simulink model "Cardio_SA_LV_EarlyVersion"  (R2021a)
settings: Solver=ode1  StartTime=0.0  StopTime=Beats  FixedStep=dt  MinStep=.001  RelTol=1e-3  EnableMultiTasking=on
PreLoadFcn:
  | %Time parameters
  | T = 0.0125;   %Duration of heartbeat (minutes)
  | Ts = 0.0050;   %Duration of systole   (minutes)
  | Stroke_volume = 70e-3;
  | Tmax = 0.0020;  %Time at which flow is max (minutes)
  | Qmax= Stroke_volume/(0.5*Ts);    %Max flow through aortic valve (liters/minute)
  | dt = .00005*T;
  | %This choice implies 20,000 timesteps per cardiac cycle
  | 
  | %Compliance and resistance parameters. Note that valve resistances are not
  | %supposed to be realistic, just small enough to be negligible
  | Csa = .00175; %Systemic arterial compliance (liters/(mmHg))
  | Rs = 17.86; %Systemic resistance (mmHg/(liters/minute))
  | Rmi = .01; %mitral valve resistance (mmHg/(liters/minute))
  | RAo = .01; %Aortic valve resistance (mmHg/(liters/minute))
  | 
  | Vlvd = .027; %Left ventricular volume when PLV = 0 (liters)
  | Vsad = .825; %Systemic arterial volume when Psa = 0 (liters)
  | Pla = 5; %Left atrial pressure (mmHg)
  | 
  | %Parameters for Clv(t)
  | CLVD = .0146; %Max (diastolic) value of CLV (liters/mmHg)
  | CLVS = .00003; %Min (systolic) value of CLV (liters/mmHg)
  | tauS = .0025; %CLV time constant during systole (minutes)
  | tauD = .001; %CLV time constant during diastole (minutes)
  | 
  | %Initialization parameters
  | Plvi = 5; %initial value of PLV (mmHg)
  | Psai = 80; %initial value of Psa (mmHg)
  | 
  | %Don't forget to plot VSA vs. PSA and VLV vs. PLV!!!!!!! The values have
  | %been exported into the matlab workspace so you can plot them yourself!
values from neighbouring files (symbols this model uses):
  AoBkflo = 0.00    (= 0)    [Command_Cardio_SA_LV.m]
settings Model: Creator=MRFIL  LastModifiedBy=claudelieber
settings SolverCC: AlgebraicLoopSolver=TrustRegion
settings DataIOCC: LimitDataPoints=on  SaveFormat=Array  SignalLoggingSaveFormat=ModelDataLogs  ReturnWorkspaceOutputs=off
settings OptimizationCC: ExpressionDepthLimit=2147483647  LifeSpan=inf
settings DebuggingCC: UnderspecifiedInitializationDetection=Classic  MergeDetectMultiDrivingBlocksExec=none  SolverPrmCheckMsg=warning  FcnCallInpInsideContextMsg=warning  StateNameClashWarn=warning  SFUnexpectedBacktrackingDiag=warning  SFNoUnconditionalDefaultTransitionDiag=warning  SFExecutionAtInitializationDiag=none  ArithmeticOperatorsInVariantConditions=warning
settings HardwareCC: ProdBitPerPointer=32  ProdBitPerSizeT=32  ProdBitPerPtrDiffT=32  ProdLargestAtomicFloat=None  ProdIntDivRoundTo=Undefined  ProdEndianess=Unspecified  ProdWordSize=32  ProdHWDeviceType=32-bit Generic
settings ModelReferenceCC: PropagateSignalLabelsOutOfModel=off
settings SFSimCC: SimUseLocalCustomCode=off  CustomCodeUndefinedFunction=UseInterfaceOnly
settings RTWCC: RTWUseLocalCustomCode=off  DLArmComputeVersion=20.02.1
settings CodeAppCC: StateflowObjectComments=on
settings GRTTargetCC: TargetLangStandard=C89/C90 (ANSI)  CombineOutputUpdateFcns=off  GRTInterface=on
settings ConfigComp: CovMetricSettings=dw  CovSaveCumulativeToWorkspaceVar=on  CovSaveSingleToWorkspaceVar=on  CovExternalEMLEnable=off

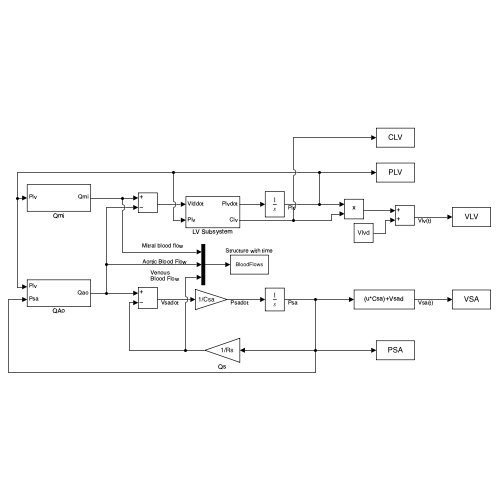
[thumbnail: Simulink's stored preview of the top-level diagram]
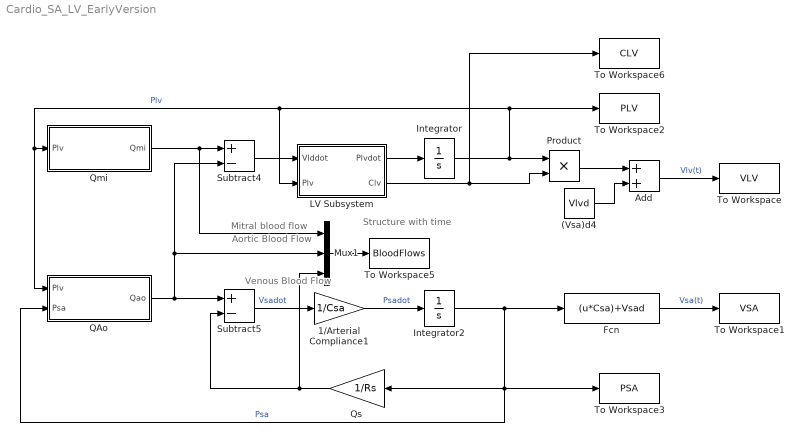
== system Cardio_SA_LV_EarlyVersion ==
  note: Structure with time
  note: Venous
      | Blood Flow
  note: Aortic Blood Flow
  note: Mitral blood flow
  (Vsa)d4 : Constant  Value=Vlvd
  1/Arterial Compliance1 : Gain  Gain=1/Csa
  Add : Sum
  Fcn : Fcn  Expr=(u*Csa)+Vsad
  Integrator : Integrator  InitialCondition=Plvi
  Integrator2 : Integrator  InitialCondition=Psai
  LV Subsystem : Subsystem
  Mux1 : Mux  Inputs=3
  Product : Product  RndMeth=Zero
  QAo : Subsystem
  Qmi : Subsystem
  Qs : Gain  Gain=1/Rs
  Subtract4 : Sum  Inputs=+-
  Subtract5 : Sum  Inputs=+-
  To Workspace : ToWorkspace  VariableName=VLV  SampleTime=-1
  To Workspace1 : ToWorkspace  VariableName=VSA  SampleTime=-1
  To Workspace2 : ToWorkspace  VariableName=PLV  SampleTime=-1
  To Workspace3 : ToWorkspace  VariableName=PSA  SampleTime=-1
  To Workspace5 : ToWorkspace  VariableName=BloodFlows  SaveFormat=Structure With Time  SampleTime=-1
  To Workspace6 : ToWorkspace  VariableName=CLV  SampleTime=-1
  wires:
  Fcn/1 -> To Workspace1/1  "Vsa(t)"
  Subtract5/1 -> 1/Arterial Compliance1/1  "Vsadot"
  1/Arterial Compliance1/1 -> Integrator2/1  "Psadot"
  Integrator2/1 -> QAo/2(Psa), To Workspace3/1, Qs/1, Fcn/1  "Psa"
  Qs/1 -> Subtract5/2, Mux1/3
  QAo/1(Qao) -> Mux1/2, Subtract4/2, Subtract5/1
  Qmi/1(Qmi) -> Subtract4/1, Mux1/1
  Product/1 -> Add/1
  (Vsa)d4/1 -> Add/2
  Add/1 -> To Workspace/1  "Vlv(t)"
  Subtract4/1 -> LV Subsystem/1(Vlddot)
  LV Subsystem/1(Plvdot) -> Integrator/1
  Integrator/1 -> Product/1, LV Subsystem/2(Plv), QAo/1(Plv), Qmi/1(Plv), To Workspace2/1  "Plv"
  LV Subsystem/2(Clv) -> To Workspace6/1, Product/2
  Mux1/1 -> To Workspace5/1

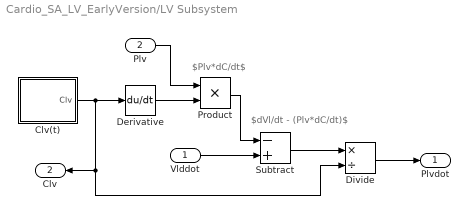
== system Cardio_SA_LV_EarlyVersion/LV Subsystem ==
  note: $dVl/dt - (Plv*dC/dt)$
  note: $Plv*dC/dt$
  Vlddot : Inport
  Plv : Inport  Port=2
  Clv(t) : Subsystem
  Derivative : Derivative
  Divide : Product  Inputs=*/
  Product : Product  RndMeth=Zero
  Subtract : Sum  Inputs=-+
  Plvdot : Outport  VectorParamsAs1DForOutWhenUnconnected=off
  Clv : Outport  Port=2  VectorParamsAs1DForOutWhenUnconnected=off
  wires:
  Clv(t)/1(Clv) -> Derivative/1, Clv/1, Divide/2
  Derivative/1 -> Product/2
  Plv/1 -> Product/1
  Product/1 -> Subtract/1
  Vlddot/1 -> Subtract/2
  Subtract/1 -> Divide/1
  Divide/1 -> Plvdot/1

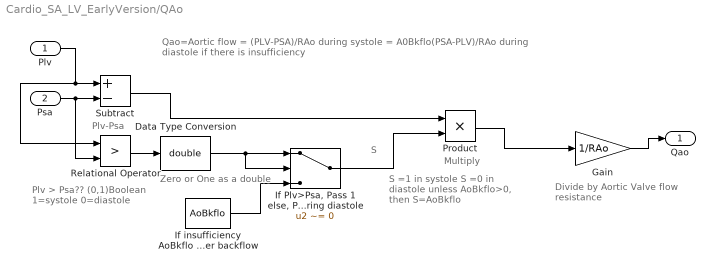
== system Cardio_SA_LV_EarlyVersion/QAo ==
  note: S
  note: S =1 in systole
      | S =0 in diastole
      | unless AoBkflo>0,
      | then S=AoBkflo
  note: Qao=Aortic flow = (PLV-PSA)/RAo during systole
      | = A0Bkflo(PSA-PLV)/RAo during diastole
      | if there is insufficiency
  note: Divide by
      | Aortic Valve
      | flow resistance
  note: Plv > Psa??
      | (0,1)Boolean
      | 1=systole
      | 0=diastole
  note: Multiply
  note: Zero or One
      | as a double
  note: Plv-Psa
  Plv : Inport
  Psa : Inport  Port=2
  Data Type Conversion : DataTypeConversion  OutDataTypeStr=double
  Gain : Gain  Gain=1/RAo
  "If Plv>Psa, Pass 1 else, Pass AoBkflo i.e. pass PLV-PSA during systole and AoBkflo*(PSA-PLV) during diastole" : Switch  Criteria=u2 ~= 0
  If insufficiency AoBkflo multiplies pressure difference during diastole divided by RAo to render backflow : Constant  Value=AoBkflo
  Product : Product  RndMeth=Zero
  Relational Operator : RelationalOperator  Operator=>  OutDataTypeStr=boolean  RndMeth=Nearest
  Subtract : Sum  Inputs=+-
  Qao : Outport  VectorParamsAs1DForOutWhenUnconnected=off
  wires:
  "If Plv>Psa, Pass 1 else, Pass AoBkflo i.e. pass PLV-PSA during systole and AoBkflo*(PSA-PLV) during diastole"/1 -> Product/2
  Relational Operator/1 -> Data Type Conversion/1
  Gain/1 -> Qao/1
  Psa/1 -> Subtract/2, Relational Operator/2
  Product/1 -> Gain/1
  Data Type Conversion/1 -> "If Plv>Psa, Pass 1 else, Pass AoBkflo i.e. pass PLV-PSA during systole and AoBkflo*(PSA-PLV) during diastole"/2, "If Plv>Psa, Pass 1 else, Pass AoBkflo i.e. pass PLV-PSA during systole and AoBkflo*(PSA-PLV) during diastole"/1
  If insufficiency AoBkflo multiplies pressure difference during diastole divided by RAo to render backflow/1 -> "If Plv>Psa, Pass 1 else, Pass AoBkflo i.e. pass PLV-PSA during systole and AoBkflo*(PSA-PLV) during diastole"/3
  Plv/1 -> Subtract/1, Relational Operator/1
  Subtract/1 -> Product/1

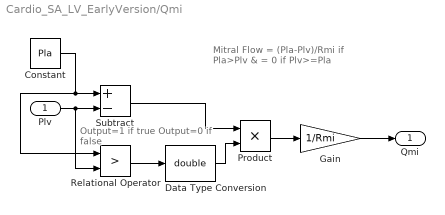
== system Cardio_SA_LV_EarlyVersion/Qmi ==
  note: Mitral Flow = (Pla-Plv)/Rmi if Pla>Plv
      | & = 0 if Plv>=Pla
  note: Output=1 if true
      | Output=0 if false
  Plv : Inport
  Constant : Constant  Value=Pla
  Data Type Conversion : DataTypeConversion  OutDataTypeStr=double
  Gain : Gain  Gain=1/Rmi
  Product : Product  RndMeth=Zero
  Relational Operator : RelationalOperator  Operator=>  OutDataTypeStr=boolean  RndMeth=Nearest
  Subtract : Sum  Inputs=+-
  Qmi : Outport  VectorParamsAs1DForOutWhenUnconnected=off
  wires:
  Constant/1 -> Relational Operator/1, Subtract/1
  Subtract/1 -> Product/1
  Product/1 -> Gain/1
  Gain/1 -> Qmi/1
  Plv/1 -> Relational Operator/2, Subtract/2
  Data Type Conversion/1 -> Product/2
  Relational Operator/1 -> Data Type Conversion/1

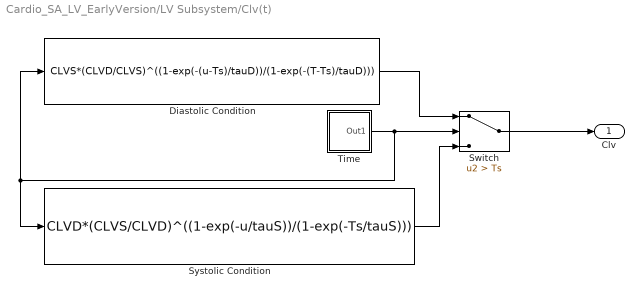
== system Cardio_SA_LV_EarlyVersion/LV Subsystem/Clv(t) ==
  Diastolic Condition : Fcn  Expr=CLVS*(CLVD/CLVS)^((1-exp(-(u-Ts)/tauD))/(1-exp(-(T-Ts)/tauD)))
  Switch : Switch  Criteria=u2 > Threshold  Threshold=Ts
  Systolic Condition : Fcn  Expr=CLVD*(CLVS/CLVD)^((1-exp(-u/tauS))/(1-exp(-Ts/tauS)))
  Time : Subsystem
  Clv : Outport  VectorParamsAs1DForOutWhenUnconnected=off
  wires:
  Time/1(Out1) -> Systolic Condition/1, Diastolic Condition/1, Switch/2
  Diastolic Condition/1 -> Switch/1
  Systolic Condition/1 -> Switch/3
  Switch/1 -> Clv/1

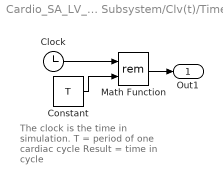
== system Cardio_SA_LV_EarlyVersion/LV Subsystem/Clv(t)/Time ==
  note: The clock is the time in simulation.
      | T = period of one cardiac cycle
      | Result = time in cycle
  Clock : Clock
  Constant : Constant  Value=T
  Math Function : Math  Operator=rem  SignedPower=on  SaturateOnIntegerOverflow=on
  Out1 : Outport  VectorParamsAs1DForOutWhenUnconnected=off
  wires:
  Math Function/1 -> Out1/1
  Constant/1 -> Math Function/2
  Clock/1 -> Math Function/1
